simulink model "state_Hinfinty"  (R2023a)
settings: Solver=VariableStepAuto  StartTime=0.0  StopTime=50  RelTol=1e-3
settings Model: Creator=belov  LastModifiedBy=belov

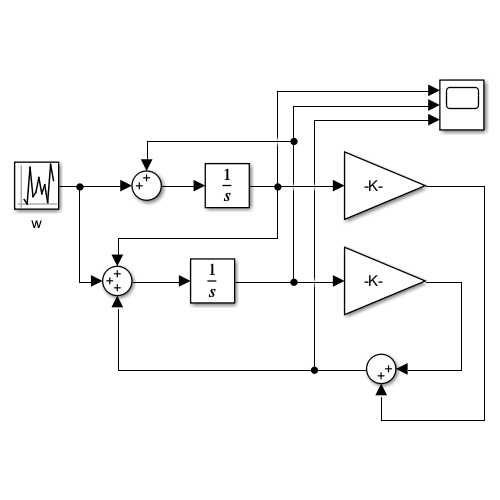
[thumbnail: Simulink's stored preview of the top-level diagram]
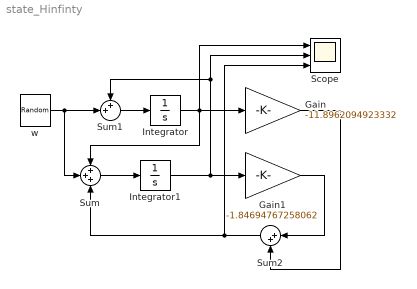
== system state_Hinfinty ==
  Gain : Gain  Gain=-11.8962094923332
  Gain1 : Gain  Gain=-1.84694767258062
  Integrator : Integrator  InitialCondition=1
  Integrator1 : Integrator  InitialCondition=-1
  Scope : Scope  NumInputPorts=3
  Sum : Sum  Inputs=+++
  Sum1 : Sum  Inputs=++|
  Sum2 : Sum  Inputs=|++
  w : UniformRandomNumber  Minimum=-0.05  Maximum=0.05  SampleTime=0.1
  wires:
  Sum/1 -> Integrator1/1
  Integrator/1 -> Sum/1, Gain/1, Scope/1
  Sum1/1 -> Integrator/1
  Integrator1/1 -> Scope/2, Sum1/1, Gain1/1
  Gain/1 -> Sum2/2
  Gain1/1 -> Sum2/1
  Sum2/1 -> Sum/3, Scope/3
  w/1 -> Sum/2, Sum1/2
